simulink model "HQEV_MiL_20160830_integrate"  (Simulink 8.3)
settings: Solver=FixedStepDiscrete  StartTime=0.0  StopTime=inf  FixedStep=0.01  RelTol=1e-3
PostLoadFcn:
  | , if any(exist('dsrtsu_mdlpostloadfcn', 'file') == [2, 3, 6]), try dsrtsu_mdlpostloadfcn('Execute', bdroot); catch fprintf('Error in PostLoadFcn (dsrtsu_mdlpostloadfcn) for model "%s":\n %s\n', bdroot, lasterr); end, end,
values from neighbouring files (symbols this model uses):
  Bat_C_Ah = 36    [parameter_V1.mat]
  Bat_ocv_xIndex = [5 10 20 30 40 50 60 70 80 90 95]    [parameter_V1.mat]
  Bat_ocv_z = [329 332 340 345 347 351 358 372 377 386 391]    [parameter_V1.mat]
  Bat_R_ohm_z = [4.41 3.46 1.57 1.07 0.76 0.63 0.55 0.44 0.41 0.4 0.4 3.14 ... (66 elements, 11x6)]    [parameter_V1.mat]
  Bat_SOC_Init = 90    [parameter_V1.mat]
  Env_hum_pct_Ambient = 30    [parameter_V1.mat]
  Env_Slope_deg = 0    [parameter_V1.mat]
  Env_Temp_degC_Ambient = 25    [parameter_V1.mat]
  Env_v_kmph_HWind = 0    [parameter_V1.mat]
  Reducer_F_i = 7.23    [parameter_V1.mat]
  Reducer_R_i = 7.23    [parameter_V1.mat]
  Veh =     [parameter_V1.mat]
  Veh_A_m2_Fr = 2.246    [parameter_V1.mat]
  Veh_F_Brake =     [parameter_V1.mat]
  Veh_fac_AirDrag = 0.326    [parameter_V1.mat]
  Veh_fac_WhDragFrict_0 = 0.011    [parameter_V1.mat]
  Veh_g_mps2_C = 9.81    [parameter_V1.mat]
  Veh_GainBrake =     [parameter_V1.mat]
  Veh_h_m_COGHigh = 0.5    [parameter_V1.mat]
  Veh_J_kgm2_Wh = 1.3635    [parameter_V1.mat]
  Veh_L_m_AxlBas = 2.63    [parameter_V1.mat]
  Veh_M_kg = 1427    [parameter_V1.mat]
  Veh_mu_Brake = 0.4    [parameter_V1.mat]
  Veh_mu_Tyre =     [parameter_V1.mat]
  Veh_num_FrictPair = 8    [parameter_V1.mat]
  Veh_pct_Brk = 70    [parameter_V1.mat]
  Veh_r_dyn =     [parameter_V1.mat]
  Veh_r_m_BrkDisk = 0.136    [parameter_V1.mat]
  Veh_rho_kgpm3_Air = 1.2258    [parameter_V1.mat]
undefined symbols (not defined in the file or in its folder): DiscIntNeverNeededParam, p_bool_False_M, p_bool_True_M
libraries: BaseOperationLib_Browser x38, simulink x9, DTQC_lib x1, ERR_lib x1, MQM_lib x1, PTCL_lib x1, PUD_lib x1, TQD_lib x1, TQR_lib x1, VMM_lib x1, ACCA_lib x1, BBCA_lib x1
(part 10 of 15)

== system HQEV_MiL_20160830_integrate/MiL/Test_Integration/HCU/HCU/HCU/EVManager/evm_core ==
  Bus_hw_prep : Inport
  Bus_hw_algo : Inport  Port=2
  Bus Creator1 : BusCreator  Inputs=7
  DTQC : Subsystem
  ERR : Subsystem
  MQM : Subsystem
  PTCL : Subsystem
  PUD : Subsystem
  TQD : Subsystem
  TQR : Subsystem
  VMM : Subsystem
  Bus_evm_core : Outport
  wires:
  ERR/1(Bus_ERR) -> VMM/4(Bus_ERR)
  TQD/1(Bus_TQD) -> Bus Creator1/5, DTQC/1(Bus_TQD)
  TQR/1(Bus_TQR) -> Bus Creator1/4, TQD/1(Bus_TQR)
  PTCL/1(Bus_PTCL) -> Bus Creator1/3, TQR/1(Bus_PTCL)
  VMM/1(Bus_VMM) -> Bus Creator1/1, PUD/3(Bus_VMM)
  PUD/1(Bus_PUD) -> Bus Creator1/2, VMM/3(Bus_PUD)
  Bus_hw_algo/1 -> DTQC/3(Bus_hw_algo), MQM/3(Bus_hw_algo), TQD/3(Bus_hw_algo), TQR/3(Bus_hw_algo), PUD/2(Bus_hw_algo), ERR/2(Bus_hw_algo), VMM/2(Bus_hw_algo)
  Bus_hw_prep/1 -> DTQC/2(Bus_hw_prep), MQM/2(Bus_hw_prep), TQD/2(Bus_hw_prep), TQR/2(Bus_hw_prep), PTCL/1(Bus_hw_prep), PUD/1(Bus_hw_prep), ERR/1(Bus_hw_prep), VMM/1(Bus_hw_prep)
  Bus Creator1/1 -> Bus_evm_core/1  "Bus_evm_core"
  DTQC/1(Bus_DTQC) -> Bus Creator1/6, MQM/1(Bus_DTQC)
  MQM/1(Bus_MQM) -> Bus Creator1/7

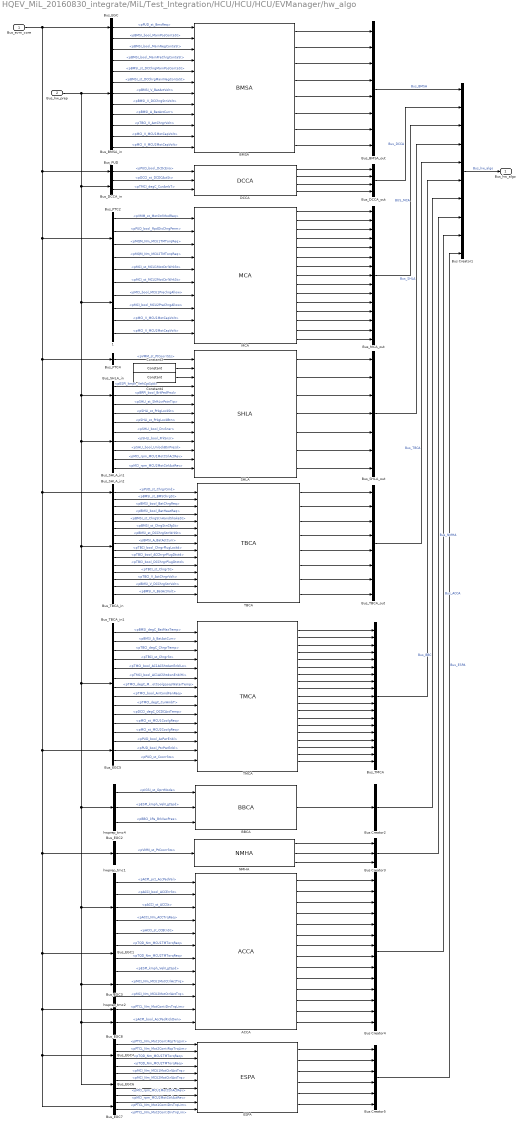
== system HQEV_MiL_20160830_integrate/MiL/Test_Integration/HCU/HCU/HCU/EVManager/hw_algo ==
  Bus_evm_core : Inport
  Bus_hw_prep : Inport  Port=2
  " 1" : BusSelector  OutputSignals=Bus_MCI.pMCI_st_MCU1MotCtrlWrkSt,Bus_MCI.pMCI_st_MCU2MotCtrlWrkSt,Bus_MCI.pMCI_bool_MCU1PrechrgAllow,Bus_MCI.pMCI_bool_MCU2PreChrgAllow,Bus_MCI.pMCI_V_MCU1MotCapVolt,Bus_MCI.pMCI_V_MCU2MotCapVolt
  ACCA : ACCA_lib/ACCA  SystemSampleTime=-1
  BBCA : BBCA_lib/BBCA  SystemSampleTime=-1
  BMSA : BMSA_lib/BMSA  SystemSampleTime=-1
  Bus Creator1 : BusCreator  Inputs=10
  Bus Creator2 : BusCreator  Inputs=1
  Bus Creator3 : BusCreator  Inputs=3
  Bus Creator4 : BusCreator  Inputs=14
  Bus Creator5 : BusCreator  Inputs=6
  Bus_BMSA_in : BusSelector  OutputSignals=Bus_BMSI.pBMSI_bool_MainPosContaSt,Bus_BMSI.pBMSI_bool_MainNegContaSt,Bus_BMSI.pBMSI_bool_MainPreChrgContaSt,Bus_BMSI.pBMSI_st_DCChrgMainPosContaSt,Bus_BMSI.pBMSI_st_DCChrgMainNegContaSt,Bus_BMSI.pBMSI_V_BatActVolt,Bus_BMSI.pBMSI_V_DCChrgStnVolt,Bus_BMSI.pBMSI_A_BatActCurr,Bus_TBCI.pTBCI_V_ActChrgrVolt,Bus_MCI.pMCI_V_MCU1MotCapVolt,Bus_MCI.pMCI_V_MCU2MotCapVolt
  Bus_BMSA_out : BusCreator  Inputs=8
  Bus_DCCA_in : BusSelector  OutputSignals=Bus_DCCI.pDCCI_st_DCDCActSt,Bus_TMCI.pTMCI_degC_CurAmbT
  Bus_DCCA_out : BusCreator
  Bus_EGC : BusSelector  OutputSignals=Bus_PUD.pPUD_st_BmsReq
  Bus_EGC1 : BusSelector  OutputSignals=Bus_TQD.pTQD_Nm_MCU1TMTorqReq,Bus_TQD.pTQD_Nm_MCU2TMTorqReq
  Bus_EGC2 : BusSelector  OutputSignals=Bus_VMM.pVMM_st_PtCoorrSts
  Bus_EGC3 : BusSelector  OutputSignals=Bus_PTCL.pPTCL_Nm_MotContiDrvTrqLim
  Bus_EGC4 : BusSelector  OutputSignals=Bus_PTCL.pPTCL_Nm_Mot1ContiRcpTrqLim,Bus_PTCL.pPTCL_Nm_Mot2ContiRcpTrqLim,Bus_TQD.pTQD_Nm_MCU1TMTorqReq,Bus_TQD.pTQD_Nm_MCU2TMTorqReq
  Bus_EGC5 : BusSelector  OutputSignals=Bus_PUD.pPUD_bool_AcPwrEnbl,Bus_PUD.pPUD_bool_PtcPwrEnbl,Bus_PUD.pPUD_st_CoorrSts
  Bus_EGC6 : BusSelector  OutputSignals=Bus_MCI.pMCI_Nm_MCU1MotCtrlActTrq,Bus_MCI.pMCI_Nm_MCU2MotCtrlActTrq,Bus_MCI.pMCI_rpm_MCU1MotCtrlActRev,Bus_MCI.pMCI_rpm_MCU2MotCtrlActRev
  Bus_EGC7 : BusSelector  OutputSignals=Bus_PTCL.pPTCL_Nm_Mot1ContiDrvTrqLim,Bus_PTCL.pPTCL_Nm_Mot2ContiDrvTrqLim
  Bus_EGC8 : BusSelector  OutputSignals=Bus_ACPI.pACPI_bool_AccPedKickDwn
  Bus_MCA_out : BusCreator  Inputs=15
  Bus_PTC2 : BusSelector  OutputSignals=Bus_VMM.pVMM_st_MotCtrlModReq,Bus_PUD.pPUD_bool_RpdDisChrgPerm,Bus_MQM.pMQM_Nm_MCU1TMTorqReq,Bus_MQM.pMQM_Nm_MCU2TMTorqReq
  Bus_PTC4 : BusSelector  OutputSignals=Bus_VMM.pVMM_st_PtCoorrSts
  Bus_PUD : BusSelector  OutputSignals=Bus_PUD.pPUD_bool_DcDcEna
  Bus_SHLA_in : BusSelector  OutputSignals=Bus_ESPI.pESPI_kmph_VehLgtSpd,Bus_BRPI.pBRPI_bool_BrkPedPrsd,Bus_SHLI.pSHLI_st_ShftLvrPstnTip
  Bus_SHLA_in1 : BusSelector  OutputSignals=Bus_SHLI.pSHLI_st_PrkgLockSt,Bus_SHLI.pSHLI_st_PrkgLockBtn,Bus_SHLI.pSHLI_bool_DrvSnsr,Bus_SHLI.pSHLI_bool_PrkSnsr,Bus_SHLI.pSHLI_bool_UnlockBtnPresd,Bus_MCI.pMCI_rpm_MCU1MotCtrlActRev,Bus_MCI.pMCI_rpm_MCU2MotCtrlActRev
  Bus_SHLA_in2 : BusSelector  OutputSignals=Bus_PUD.pPUD_st_ChrgrCmd
  Bus_SHLA_out : BusCreator  Inputs=7
  Bus_TBCA_in : BusSelector  OutputSignals=Bus_BMSI.pBMSI_st_BMSChrgSt,Bus_BMSI.pBMSI_bool_BatChrgReq,Bus_BMSI.pBMSI_bool_BatHeatReq,Bus_BMSI.pBMSI_st_ChrgStnHandShakeSt,Bus_BMSI.pBMSI_st_ChrgStnCfgSt,Bus_BMSI.pBMSI_st_DCChrgStnWrkSt,Bus_BMSI.pBMSI_A_BatActCurr,Bus_TBCI.pTBCI_bool_ChrgrPlugLockd,Bus_TBCI.pTBCI_bool_ACChrgrPlugDtctd,Bus_TBCI.pTBCI_bool_DCChrgrPlugDtctd,Bus_TBCI.pTBCI_st_ChrgrSt,Bus_TBCI.pTBCI_V_ActChrgrVolt,Bus_BMSI.pBMSI_V_DCChrgStnVolt,Bus_BMSI.pBMSI_V_BatActVolt
  Bus_TBCA_in1 : BusSelector  OutputSignals=Bus_BMSI.pBMSI_degC_BatMaxTemp,Bus_BMSI.pBMSI_A_BatActCurr,Bus_TBCI.pTBCI_degC_ChrgrTemp,Bus_TBCI.pTBCI_st_ChrgrSt,Bus_TMCI.pTMCI_bool_AC1ACShtdwnEnblLo,Bus_TMCI.pTMCI_bool_AC1ACShtdwnEnblHi,Bus_TMCI.pTMCI_degC_MotCoolgLoopWaterTemp,Bus_TMCI.pTMCI_bool_AirCondFanReq,Bus_TMCI.pTMCI_degC_CurAmbT,Bus_DCCI.pDCCI_degC_DCDCActTemp,Bus_MCI.pMCI_st_MCU1CoolgReq,Bus_MCI.pMCI_st_MCU2CoolgReq
  Bus_TBCA_out : BusCreator  Inputs=8
  Bus_TMCA : BusCreator  Inputs=19
  Constant3 : BaseOperationLib_Browser/Sources&Sinks/Constant  Value=p_bool_True_M  OutMin=[]  OutMax=[]  OutDataTypeMode=boolean  OutDataType=fixdt(1, 16)  ConRadixGroup=Use specified scaling  OutScaling=2^0  OutDataTypeStr=boolean
  Constant4 : BaseOperationLib_Browser/Sources&Sinks/Constant  Value=p_bool_False_M  OutMin=[]  OutMax=[]  OutDataTypeMode=boolean  OutDataType=fixdt(1, 16)  ConRadixGroup=Use specified scaling  OutScaling=2^0  OutDataTypeStr=boolean
  DCCA : DCCA_lib/DCCA  SystemSampleTime=-1
  ESPA : ESPA_lib/ESPA  SystemSampleTime=-1
  MCA : MCA_lib/MCA  SystemSampleTime=-1
  NMHA : NMHA_lib/NMHA  SystemSampleTime=-1
  SHLA : SHLA_lib/SHLA  SystemSampleTime=-1
  TBCA : TBCA_lib/TBCA  SystemSampleTime=-1
  TMCA : TMCA_lib/TMCA  SystemSampleTime=-1
  hwprep_tmc1 : BusSelector  OutputSignals=Bus_ACPI.pACPI_pct_AccPedVal,Bus_ACCI.pACCI_bool_ACCErrSt,Bus_ACCI.pACCI_st_ACCSt,Bus_ACCI.pACCI_Nm_ACCTrqReq,Bus_ACCI.pACCI_st_CCBtnSt
  hwprep_tmc2 : BusSelector  OutputSignals=Bus_ESPI.pESPI_kmph_VehLgtSpd,Bus_MCI.pMCI_Nm_MCU1MotCtrlActTrq,Bus_MCI.pMCI_Nm_MCU2MotCtrlActTrq
  hwprep_tmc4 : BusSelector  OutputSignals=Bus_IGSI.pIGSI_st_OprtMode,Bus_ESPI.pESPI_kmph_VehLgtSpd,Bus_BBCI.pBBCI_kPa_BrkVacPres
  Bus_hw_algo : Outport
  wires:
  Bus_BMSA_in/8 -> BMSA/9  "<pBMSI_A_BatActCurr>"
  MCA/15 -> Bus_MCA_out/15
  MCA/14 -> Bus_MCA_out/14
  MCA/13 -> Bus_MCA_out/13
  MCA/12 -> Bus_MCA_out/12
  MCA/11 -> Bus_MCA_out/11
  MCA/10 -> Bus_MCA_out/10
  MCA/9 -> Bus_MCA_out/9
  MCA/8 -> Bus_MCA_out/8
  MCA/7 -> Bus_MCA_out/7
  MCA/6 -> Bus_MCA_out/6
  MCA/5 -> Bus_MCA_out/5
  MCA/4 -> Bus_MCA_out/4
  MCA/3 -> Bus_MCA_out/3
  MCA/2 -> Bus_MCA_out/2
  MCA/1 -> Bus_MCA_out/1
  DCCA/1 -> Bus_DCCA_out/1
  Bus_DCCA_in/1 -> DCCA/2  "<pDCCI_st_DCDCActSt>"
  Bus_PUD/1 -> DCCA/1  "<pPUD_bool_DcDcEna>"
  DCCA/2 -> Bus_DCCA_out/2
  DCCA/3 -> Bus_DCCA_out/3
  DCCA/4 -> Bus_DCCA_out/4
  Bus_DCCA_in/2 -> DCCA/3  "<pTMCI_degC_CurAmbT>"
  Bus_DCCA_out/1 -> Bus Creator1/2  "Bus_DCCA"
  Constant4/1 -> SHLA/3
  Constant3/1 -> SHLA/2
  Bus_SHLA_in1/7 -> SHLA/13  "<pMCI_rpm_MCU2MotCtrlActRev>"
  Bus_SHLA_in1/6 -> SHLA/12  "<pMCI_rpm_MCU1MotCtrlActRev>"
  Bus_PTC2/2 -> MCA/2  "<pPUD_bool_RpdDisChrgPerm>"
  SHLA/7 -> Bus_SHLA_out/7
  SHLA/6 -> Bus_SHLA_out/6
  SHLA/5 -> Bus_SHLA_out/5
  SHLA/4 -> Bus_SHLA_out/4
  SHLA/3 -> Bus_SHLA_out/3
  SHLA/2 -> Bus_SHLA_out/2
  SHLA/1 -> Bus_SHLA_out/1
  Bus_SHLA_in1/5 -> SHLA/11  "<pSHLI_bool_UnlockBtnPresd>"
  Bus_SHLA_in/3 -> SHLA/6  "<pSHLI_st_ShftLvrPstnTip>"
  Bus_SHLA_in/2 -> SHLA/5  "<pBRPI_bool_BrkPedPrsd>"
  Bus_SHLA_in/1 -> SHLA/4  "<pESPI_kmph_VehLgtSpd>"
  Bus_TBCA_in/13 -> TBCA/14  "<pBMSI_V_DCChrgStnVolt>"
  Bus_TBCA_in/12 -> TBCA/13  "<pTBCI_V_ActChrgrVolt>"
  Bus Creator3/1 -> Bus Creator1/8  "Bus_NMHA"
  NMHA/3 -> Bus Creator3/3
  NMHA/2 -> Bus Creator3/2
  NMHA/1 -> Bus Creator3/1
  Bus_EGC2/1 -> NMHA/1  "<pVMM_st_PtCoorrSts>"
  Bus_PTC2/4 -> MCA/4  "<pMQM_Nm_MCU2TMTorqReq>"
  Bus_PTC2/3 -> MCA/3  "<pMQM_Nm_MCU1TMTorqReq>"
  Bus_PTC2/1 -> MCA/1  "<pVMM_st_MotCtrlModReq>"
  Bus_TBCA_in/7 -> TBCA/8  "<pBMSI_A_BatActCurr>"
  BMSA/8 -> Bus_BMSA_out/8
  BMSA/7 -> Bus_BMSA_out/7
  BMSA/6 -> Bus_BMSA_out/6
  BMSA/5 -> Bus_BMSA_out/5
  BMSA/4 -> Bus_BMSA_out/4
  BMSA/3 -> Bus_BMSA_out/3
  BMSA/2 -> Bus_BMSA_out/2
  BMSA/1 -> Bus_BMSA_out/1
  Bus_BMSA_in/11 -> BMSA/12  "<pMCI_V_MCU2MotCapVolt>"
  Bus_BMSA_in/10 -> BMSA/11  "<pMCI_V_MCU1MotCapVolt>"
  Bus_BMSA_in/9 -> BMSA/10  "<pTBCI_V_ActChrgrVolt>"
  Bus_BMSA_in/7 -> BMSA/8  "<pBMSI_V_DCChrgStnVolt>"
  hwprep_tmc4/3 -> BBCA/3  "<pBBCI_kPa_BrkVacPres>"
  Bus Creator2/1 -> Bus Creator1/7  "Bus_BBC"
  hwprep_tmc4/1 -> BBCA/1  "<pIGSI_st_OprtMode>"
  hwprep_tmc4/2 -> BBCA/2  "<pESPI_kmph_VehLgtSpd>"
  BBCA/1 -> Bus Creator2/1
  Bus_MCA_out/1 -> Bus Creator1/3  "BUS_MCA"
  " 1"/6 -> MCA/10  "<pMCI_V_MCU2MotCapVolt>"
  " 1"/5 -> MCA/9  "<pMCI_V_MCU1MotCapVolt>"
  " 1"/1 -> MCA/5  "<pMCI_st_MCU1MotCtrlWrkSt>"
  " 1"/4 -> MCA/8  "<pMCI_bool_MCU2PreChrgAllow>"
  " 1"/3 -> MCA/7  "<pMCI_bool_MCU1PrechrgAllow>"
  " 1"/2 -> MCA/6  "<pMCI_st_MCU2MotCtrlWrkSt>"
  Bus_TBCA_in/11 -> TBCA/12  "<pTBCI_st_ChrgrSt>"
  TBCA/8 -> Bus_TBCA_out/8
  Bus_EGC/1 -> BMSA/1  "<pPUD_st_BmsReq>"
  Bus_BMSA_in/6 -> BMSA/7  "<pBMSI_V_BatActVolt>"
  Bus_BMSA_in/5 -> BMSA/6  "<pBMSI_st_DCChrgMainNegContaSt>"
  Bus_BMSA_in/4 -> BMSA/5  "<pBMSI_st_DCChrgMainPosContaSt>"
  Bus_BMSA_in/3 -> BMSA/4  "<pBMSI_bool_MainPreChrgContaSt>"
  Bus_BMSA_in/2 -> BMSA/3  "<pBMSI_bool_MainNegContaSt>"
  Bus_BMSA_in/1 -> BMSA/2  "<pBMSI_bool_MainPosContaSt>"
  Bus_TBCA_in/10 -> TBCA/11  "<pTBCI_bool_DCChrgrPlugDtctd>"
  Bus_TBCA_in/9 -> TBCA/10  "<pTBCI_bool_ACChrgrPlugDtctd>"
  Bus_TBCA_in/8 -> TBCA/9  "<pTBCI_bool_ChrgrPlugLockd>"
  Bus_TBCA_in/6 -> TBCA/7  "<pBMSI_st_DCChrgStnWrkSt>"
  Bus_TBCA_in/5 -> TBCA/6  "<pBMSI_st_ChrgStnCfgSt>"
  Bus_TBCA_in/4 -> TBCA/5  "<pBMSI_st_ChrgStnHandShakeSt>"
  Bus_TBCA_in/3 -> TBCA/4  "<pBMSI_bool_BatHeatReq>"
  Bus_TBCA_in/2 -> TBCA/3  "<pBMSI_bool_BatChrgReq>"
  Bus_TBCA_in/1 -> TBCA/2  "<pBMSI_st_BMSChrgSt>"
  Bus_SHLA_in2/1 -> TBCA/1  "<pPUD_st_ChrgrCmd>"
  TBCA/7 -> Bus_TBCA_out/7
  TBCA/6 -> Bus_TBCA_out/6
  TBCA/5 -> Bus_TBCA_out/5
  TBCA/4 -> Bus_TBCA_out/4
  TBCA/3 -> Bus_TBCA_out/3
  TBCA/2 -> Bus_TBCA_out/2
  TBCA/1 -> Bus_TBCA_out/1
  Bus Creator1/1 -> Bus_hw_algo/1  "Bus_hw_algo"
  Bus_hw_prep/1 -> Bus_SHLA_in/1, Bus_SHLA_in1/1, Bus_TBCA_in1/1, hwprep_tmc4/1, hwprep_tmc1/1, hwprep_tmc2/1, Bus_EGC6/1, Bus_EGC8/1, Bus_TBCA_in/1, " 1"/1, Bus_DCCA_in/1, Bus_BMSA_in/1
  Bus_evm_core/1 -> Bus_PTC4/1, Bus_EGC5/1, Bus_EGC2/1, Bus_EGC1/1, Bus_EGC3/1, Bus_EGC4/1, Bus_EGC7/1, Bus_SHLA_in2/1, Bus_PTC2/1, Bus_PUD/1, Bus_EGC/1
  Bus_BMSA_out/1 -> Bus Creator1/1  "Bus_BMSA"
  Bus_SHLA_out/1 -> Bus Creator1/4  "Bus_SHLA"
  Bus_TBCA_out/1 -> Bus Creator1/5  "Bus_TBCA"
  Bus_SHLA_in1/1 -> SHLA/7  "<pSHLI_st_PrkgLockSt>"
  Bus_SHLA_in1/2 -> SHLA/8  "<pSHLI_st_PrkgLockBtn>"
  Bus_SHLA_in1/3 -> SHLA/9  "<pSHLI_bool_DrvSnsr>"
  Bus_SHLA_in1/4 -> SHLA/10  "<pSHLI_bool_PrkSnsr>"
  Bus_PTC4/1 -> SHLA/1  "<pVMM_st_PtCoorrSts>"
  Bus_TBCA_in/14 -> TBCA/15  "<pBMSI_V_BatActVolt>"
  TMCA/19 -> Bus_TMCA/19
  TMCA/18 -> Bus_TMCA/18
  TMCA/17 -> Bus_TMCA/17
  TMCA/16 -> Bus_TMCA/16
  TMCA/15 -> Bus_TMCA/15
  TMCA/14 -> Bus_TMCA/14
  TMCA/13 -> Bus_TMCA/13
  TMCA/12 -> Bus_TMCA/12
  TMCA/11 -> Bus_TMCA/11
  TMCA/10 -> Bus_TMCA/10
  TMCA/9 -> Bus_TMCA/9
  TMCA/8 -> Bus_TMCA/8
  TMCA/7 -> Bus_TMCA/7
  TMCA/6 -> Bus_TMCA/6
  TMCA/5 -> Bus_TMCA/5
  TMCA/4 -> Bus_TMCA/4
  TMCA/3 -> Bus_TMCA/3
  TMCA/2 -> Bus_TMCA/2
  TMCA/1 -> Bus_TMCA/1
  Bus_EGC5/3 -> TMCA/15  "<pPUD_st_CoorrSts>"
  Bus_EGC5/2 -> TMCA/14  "<pPUD_bool_PtcPwrEnbl>"
  Bus_EGC5/1 -> TMCA/13  "<pPUD_bool_AcPwrEnbl>"
  Bus_TBCA_in1/12 -> TMCA/12  "<pMCI_st_MCU2CoolgReq>"
  Bus_TBCA_in1/11 -> TMCA/11  "<pMCI_st_MCU1CoolgReq>"
  Bus_TBCA_in1/10 -> TMCA/10  "<pDCCI_degC_DCDCActTemp>"
  Bus_TBCA_in1/9 -> TMCA/9  "<pTMCI_degC_CurAmbT>"
  Bus_TBCA_in1/8 -> TMCA/8  "<pTMCI_bool_AirCondFanReq>"
  Bus_TBCA_in1/7 -> TMCA/7  "<pTMCI_degC_MotCoolgLoopWaterTemp>"
  Bus_TBCA_in1/6 -> TMCA/6  "<pTMCI_bool_AC1ACShtdwnEnblHi>"
  Bus_TBCA_in1/5 -> TMCA/5  "<pTMCI_bool_AC1ACShtdwnEnblLo>"
  Bus_TBCA_in1/4 -> TMCA/4  "<pTBCI_st_ChrgrSt>"
  Bus_TBCA_in1/3 -> TMCA/3  "<pTBCI_degC_ChrgrTemp>"
  Bus_TBCA_in1/2 -> TMCA/2  "<pBMSI_A_BatActCurr>"
  Bus_TBCA_in1/1 -> TMCA/1  "<pBMSI_degC_BatMaxTemp>"
  Bus_TMCA/1 -> Bus Creator1/6
  ACCA/1 -> Bus Creator4/1
  ACCA/2 -> Bus Creator4/2
  ACCA/3 -> Bus Creator4/3
  ACCA/4 -> Bus Creator4/4
  ACCA/5 -> Bus Creator4/5
  ACCA/6 -> Bus Creator4/6
  ACCA/7 -> Bus Creator4/7
  ACCA/8 -> Bus Creator4/8
  ACCA/9 -> Bus Creator4/9
  ACCA/10 -> Bus Creator4/10
  ACCA/11 -> Bus Creator4/11
  ACCA/12 -> Bus Creator4/12
  hwprep_tmc1/1 -> ACCA/1  "<pACPI_pct_AccPedVal>"
  hwprep_tmc1/2 -> ACCA/2  "<pACCI_bool_ACCErrSt>"
  hwprep_tmc1/3 -> ACCA/3  "<pACCI_st_ACCSt>"
  hwprep_tmc1/4 -> ACCA/4  "<pACCI_Nm_ACCTrqReq>"
  hwprep_tmc1/5 -> ACCA/5  "<pACCI_st_CCBtnSt>"
  hwprep_tmc2/1 -> ACCA/8  "<pESPI_kmph_VehLgtSpd>"
  hwprep_tmc2/2 -> ACCA/9  "<pMCI_Nm_MCU1MotCtrlActTrq>"
  hwprep_tmc2/3 -> ACCA/10  "<pMCI_Nm_MCU2MotCtrlActTrq>"
  Bus_EGC3/1 -> ACCA/11  "<pPTCL_Nm_MotContiDrvTrqLim>"
  Bus Creator4/1 -> Bus Creator1/9  "Bus_ACCA"
  ESPA/1 -> Bus Creator5/1
  ESPA/2 -> Bus Creator5/2
  ESPA/3 -> Bus Creator5/3
  ESPA/4 -> Bus Creator5/4
  Bus Creator5/1 -> Bus Creator1/10  "Bus_ESPA"
  Bus_EGC6/1 -> ESPA/5  "<pMCI_Nm_MCU1MotCtrlActTrq>"
  Bus_EGC6/2 -> ESPA/6  "<pMCI_Nm_MCU2MotCtrlActTrq>"
  Bus_EGC6/3 -> ESPA/7  "<pMCI_rpm_MCU1MotCtrlActRev>"
  Bus_EGC6/4 -> ESPA/8  "<pMCI_rpm_MCU2MotCtrlActRev>"
  ACCA/13 -> Bus Creator4/13
  ESPA/5 -> Bus Creator5/5
  ESPA/6 -> Bus Creator5/6
  Bus_EGC7/1 -> ESPA/9  "<pPTCL_Nm_Mot1ContiDrvTrqLim>"
  Bus_EGC7/2 -> ESPA/10  "<pPTCL_Nm_Mot2ContiDrvTrqLim>"
  Bus_EGC4/1 -> ESPA/1  "<pPTCL_Nm_Mot1ContiRcpTrqLim>"
  Bus_EGC4/2 -> ESPA/2  "<pPTCL_Nm_Mot2ContiRcpTrqLim>"
  Bus_EGC4/3 -> ESPA/3  "<pTQD_Nm_MCU1TMTorqReq>"
  Bus_EGC4/4 -> ESPA/4  "<pTQD_Nm_MCU2TMTorqReq>"
  Bus_EGC8/1 -> ACCA/12  "<pACPI_bool_AccPedKickDwn>"
  ACCA/14 -> Bus Creator4/14
  Bus_EGC1/1 -> ACCA/6  "<pTQD_Nm_MCU1TMTorqReq>"
  Bus_EGC1/2 -> ACCA/7  "<pTQD_Nm_MCU2TMTorqReq>"

== system HQEV_MiL_20160830_integrate/MiL/Test_Integration/HCU/HCU/HCU/EVManager/hw_post ==
  Bus_evm_core : Inport
  Bus_hw_algo : Inport  Port=2
  Bus_hw_prep : Inport  Port=3
  Bus Selector1 : BusSelector  OutputSignals=Bus_BMSA.pBMSA_bool_MaiPosContaCmd,Bus_BMSA.pBMSA_bool_MaiNegContaCmd,Bus_BMSA.pBMSA_bool_MaiPrecContaCmd,Bus_BMSA.pBMSA_bool_DCChrgNegContaCmd,Bus_BMSA.pBMSA_bool_DCChrgPosContaCmd,Bus_TBCA.pTBCA_bool_BatChrgPerm,Bus_TBCA.pTBCA_bool_BatHeatPerm,Bus_DCCA.pDCCA_bool_DcDcCmd,Bus_DCCA.pDCCA_V_DcDcOutUSp
  Bus Selector11 : BusSelector  OutputSignals=Bus_BMSI.pBMSI_st_BatIslaMeasSt,Bus_DCCI.pDCCI_st_DCDCActSt,Bus_BMSI.pBMSI_degC_BatAvgTemp,Bus_BMSI.pBMSI_st_BMSErr,Bus_BMSI.pBMSI_min_RemainChrgTime,Bus_BMSI.pBMSI_kw_InstnsPwrCnsmp,Bus_BMSI.pBMSI_V_BatActVolt
  Bus Selector12 : BusSelector  OutputSignals=Bus_VMM.pVMM_st_PtCoorrSts
  Bus Selector15 : BusSelector  OutputSignals=Bus_ESPI.pESPI_kmph_VehLgtSpd,Bus_TBCI.pTBCI_bool_ACChrgrPlugDtctd,Bus_TBCI.pTBCI_bool_DCChrgrPlugDtctd,Bus_ARBI.pARBI_st_StCrash
  Bus Selector19 : BusSelector  OutputSignals=signal6.pTMCA_bool_RemainACOnTip,Bus_NMHA.pNMHA_bool_CanSlpCmd,BUS_MCA.pMCA_Nm_MCU1TMTorqReq,BUS_MCA.pMCA_Nm_MCU2TMTorqReq
  Bus Selector2 : BusSelector  OutputSignals=Bus_ACPI.pACPI_pct_AccPedVal,Bus_BRPI.pBRPI_bool_BrkPedPrsd
  Bus Selector3 : BusSelector  OutputSignals=Bus_ACCA.pACCA_bool_KickDwnReq,Bus_ACCA.pACCA_bool_AccelPedOvrid,Bus_ACCA.pACCA_pct_CalcAccelPedPstn,Bus_ACCA.pACCA_bool_RespACC,Bus_ACCA.pACCA_bool_CCMainSwt,Bus_ACCA.pACCA_bool_CCCancelSwt,Bus_ACCA.pACCA_bool_CCSetOrCoastSwt,Bus_ACCA.pACCA_bool_HeadwaySwt,Bus_ACCA.pACCA_bool_CCSwtErr,Bus_ACCA.pACCA_bool_CCRsmOrAccelSwt,Bus_ACCA.pACCA_Nm_ActDrvReqTrq,Bus_ACCA.pACCA_Nm_MotMaxDrvTrq,Bus_ACCA.pACCA_Nm_IndicateDrvPrimTrq,Bus_ACCA.pACCA_Nm_IndicateDrvSecTrq
  Bus Selector30 : BusSelector  OutputSignals=Bus_VMM.pVMM_st_PtCoorrSts
  Bus Selector32 : BusSelector  OutputSignals=Bus_BMSI.pBMSI_A_BatActCurr,Bus_TBCI.pTBCI_bool_ACChrgrPlugDtctd,Bus_TBCI.pTBCI_bool_DCChrgrPlugDtctd,Bus_BMSI.pBMSI_st_BMSChrgSt,Bus_BMSI.pBMSI_pct_BatSOC,Bus_SHLI.pSHLI_st_ECOSwtSt,Bus_IGSI.pIGSI_st_OprtMode,Bus_MCI.pMCI_Nm_MCU1MotCtrlActTrq,Bus_MCI.pMCI_rpm_MCU1MotCtrlActRev,Bus_MCI.pMCI_rpm_MCU2MotCtrlActRev,Bus_DCCI.pDCCI_V_DCDCOutVolt
  Bus Selector33 : BusSelector  OutputSignals=BUS_MCA.pMCA_Nm_MCU1TMTorqReq,BUS_MCA.pMCA_bool_MCU1MotRpdDchaReq,BUS_MCA.pMCA_st_MCU1MotCtlrStModReq,BUS_MCA.pMCA_bool_MCU1AntijerkOffReq,BUS_MCA.pMCA_bool_MCU1StopReqToMCU,BUS_MCA.pMCA_Nm_MCU2TMTorqReq,BUS_MCA.pMCA_bool_MCU2MotRpdDchaReq,BUS_MCA.pMCA_st_MCU2MotCtlrStModReq,BUS_MCA.pMCA_bool_MCU2AntijerkOffReq,BUS_MCA.pMCA_bool_MCU2StopReqToMCU,Bus_NMHA.pNMHA_bool_CanSlpCmd
  Bus Selector34 : BusSelector  OutputSignals=Bus_BBC.pBBCA_bool_BrkVacPmpCmd,signal6.pTMCA_pct_PtcCtrlCmd,signal6.pTMCA_bool_HiSpdFanCmd,signal6.pTMCA_bool_LoSpdFanCmd,signal6.pTMCA_pct_Mot1WtrPmpCmd,signal6.pTMCA_pct_BatWtrPmpCmd,signal6.pTMCA_pct_Mot2WtrPmpCmd,BUS_MCA.pMCA_bool_MotVirtIgOn,Bus_NMHA.pNMHA_bool_MaiRlyCtlCmd,Bus_NMHA.pNMHA_bool_VCUSleep,signal6.pTMCA_bool_ChargerValve1CtrlB,signal6.pTMCA_bool_ChargerValve1CtrlC,signal6.pTMCA_bool_RMotorValve2CtrlB,signal6.pTMCA_bool_RMotorValve2CtrlC
  Bus Selector4 : BusSelector  OutputSignals=Bus_ESPA.pESPA_Nm_MCU1ActBrkTrq,Bus_ESPA.pESPA_Nm_MCU1MaxDrvTrq,Bus_ESPA.pESPA_Nm_MCU1MaxGenrTrq,Bus_ESPA.pESPA_Nm_MCU2ActBrkTrq,Bus_ESPA.pESPA_Nm_MCU2MaxDrvTrq,Bus_ESPA.pESPA_Nm_MCU2MaxGenrTrq
  Bus Selector5 : BusSelector  OutputSignals=signal6.pTMCA_bool_VechPermit,signal6.pTMCA_bool_IGOffReq,signal6.pTMCA_bool_AirCdnCmd,signal6.pTMCA_bool_BatCoolgReq,Bus_SHLA.pSHLA_st_ShftLvrPosnIC,Bus_SHLA.pSHLA_st_PrkgLock
  Bus Selector6 : BusSelector  OutputSignals=Bus_ESPI.pESPI_ratio_AltitudeFac
  CAN_EV : CAN_EV_lib/CAN_EV  SystemSampleTime=-1
  CAN_PT : CAN_PT_lib/CAN_PT  SystemSampleTime=-1
  HWO : HWO_lib/HWO  SystemSampleTime=-1
  bus_CAN_EV : BusCreator  Inputs=24
  bus_CAN_PT : BusCreator  Inputs=63
  bus_HWO : BusCreator  Inputs=14
  bus_in5 : BusCreator  Inputs=3
  Bus_RTE_out : Outport
  wires:
  Bus Selector34/10 -> HWO/10  "<pNMHA_bool_VCUSleep>"
  CAN_EV/24 -> bus_CAN_EV/24
  Bus Selector33/11 -> CAN_EV/11  "<pNMHA_bool_CanSlpCmd>"
  CAN_EV/23 -> bus_CAN_EV/23
  CAN_EV/22 -> bus_CAN_EV/22
  CAN_EV/21 -> bus_CAN_EV/21
  CAN_EV/20 -> bus_CAN_EV/20
  CAN_EV/19 -> bus_CAN_EV/19
  CAN_EV/18 -> bus_CAN_EV/18
  Bus Selector15/4 -> CAN_EV/25  "<pARBI_st_StCrash>"
  Bus Selector34/1 -> HWO/1  "<pBBCA_bool_BrkVacPmpCmd>"
  bus_HWO/1 -> bus_in5/3  "HWO_BUS"
  HWO/14 -> bus_HWO/14
  HWO/13 -> bus_HWO/13
  HWO/12 -> bus_HWO/12
  HWO/11 -> bus_HWO/11
  HWO/10 -> bus_HWO/10
  HWO/9 -> bus_HWO/9
  HWO/8 -> bus_HWO/8
  HWO/7 -> bus_HWO/7
  HWO/6 -> bus_HWO/6
  HWO/5 -> bus_HWO/5
  HWO/4 -> bus_HWO/4
  HWO/3 -> bus_HWO/3
  HWO/2 -> bus_HWO/2
  HWO/1 -> bus_HWO/1
  Bus Selector34/14 -> HWO/14  "<pTMCA_bool_RMotorValve2CtrlC>"
  Bus Selector34/13 -> HWO/13  "<pTMCA_bool_RMotorValve2CtrlB>"
  Bus Selector34/12 -> HWO/12  "<pTMCA_bool_ChargerValve1CtrlC>"
  Bus Selector34/11 -> HWO/11  "<pTMCA_bool_ChargerValve1CtrlB>"
  Bus Selector34/2 -> HWO/2  "<pTMCA_pct_PtcCtrlCmd>"
  Bus Selector34/3 -> HWO/3  "<pTMCA_bool_HiSpdFanCmd>"
  Bus Selector34/4 -> HWO/4  "<pTMCA_bool_LoSpdFanCmd>"
  Bus Selector34/5 -> HWO/5  "<pTMCA_pct_Mot1WtrPmpCmd>"
  Bus Selector34/6 -> HWO/6  "<pTMCA_pct_BatWtrPmpCmd>"
  Bus Selector34/8 -> HWO/8  "<pMCA_bool_MotVirtIgOn>"
  Bus Selector34/7 -> HWO/7  "<pTMCA_pct_Mot2WtrPmpCmd>"
  Bus Selector34/9 -> HWO/9  "<pNMHA_bool_MaiRlyCtlCmd>"
  Bus Selector15/3 -> CAN_EV/24  "<pTBCI_bool_DCChrgrPlugDtctd>"
  Bus Selector15/2 -> CAN_EV/23  "<pTBCI_bool_ACChrgrPlugDtctd>"
  Bus_hw_prep/1 -> Bus Selector15/1, Bus Selector32/1, Bus Selector11/1, Bus Selector6/1, Bus Selector2/1
  Bus Selector15/1 -> CAN_EV/22  "<pESPI_kmph_VehLgtSpd>"
  Bus Selector12/1 -> CAN_EV/21  "<pVMM_st_PtCoorrSts>"
  Bus_evm_core/1 -> Bus Selector30/1, Bus Selector12/1
  Bus_hw_algo/1 -> Bus Selector19/1, Bus Selector3/1, Bus Selector34/1, Bus Selector4/1, Bus Selector5/1, Bus Selector1/1, Bus Selector33/1
  bus_in5/1 -> Bus_RTE_out/1  "Bus_RTE_out"
  bus_CAN_PT/1 -> bus_in5/2  "CAN_PT_BUS"
  bus_CAN_EV/1 -> bus_in5/1  "CAN_EV_BUS"
  CAN_EV/1 -> bus_CAN_EV/1
  CAN_EV/2 -> bus_CAN_EV/2
  CAN_EV/3 -> bus_CAN_EV/3
  CAN_EV/4 -> bus_CAN_EV/4
  CAN_EV/5 -> bus_CAN_EV/5
  CAN_EV/6 -> bus_CAN_EV/6
  CAN_EV/7 -> bus_CAN_EV/7
  CAN_EV/8 -> bus_CAN_EV/8
  CAN_EV/9 -> bus_CAN_EV/9
  CAN_EV/10 -> bus_CAN_EV/10
  CAN_EV/11 -> bus_CAN_EV/11
  CAN_EV/12 -> bus_CAN_EV/12
  CAN_EV/13 -> bus_CAN_EV/13
  CAN_EV/14 -> bus_CAN_EV/14
  CAN_EV/15 -> bus_CAN_EV/15
  CAN_EV/16 -> bus_CAN_EV/16
  CAN_EV/17 -> bus_CAN_EV/17
  Bus Selector33/1 -> CAN_EV/1  "<pMCA_Nm_MCU1TMTorqReq>"
  Bus Selector33/2 -> CAN_EV/2  "<pMCA_bool_MCU1MotRpdDchaReq>"
  Bus Selector33/3 -> CAN_EV/3  "<pMCA_st_MCU1MotCtlrStModReq>"
  Bus Selector33/4 -> CAN_EV/4  "<pMCA_bool_MCU1AntijerkOffReq>"
  Bus Selector33/5 -> CAN_EV/5  "<pMCA_bool_MCU1StopReqToMCU>"
  Bus Selector33/6 -> CAN_EV/6  "<pMCA_Nm_MCU2TMTorqReq>"
  Bus Selector33/7 -> CAN_EV/7  "<pMCA_bool_MCU2MotRpdDchaReq>"
  Bus Selector33/8 -> CAN_EV/8  "<pMCA_st_MCU2MotCtlrStModReq>"
  Bus Selector33/9 -> CAN_EV/9  "<pMCA_bool_MCU2AntijerkOffReq>"
  Bus Selector33/10 -> CAN_EV/10  "<pMCA_bool_MCU2StopReqToMCU>"
  Bus Selector1/1 -> CAN_EV/12  "<pBMSA_bool_MaiPosContaCmd>"
  Bus Selector1/2 -> CAN_EV/13  "<pBMSA_bool_MaiNegContaCmd>"
  Bus Selector1/3 -> CAN_EV/14  "<pBMSA_bool_MaiPrecContaCmd>"
  Bus Selector1/4 -> CAN_EV/15  "<pBMSA_bool_DCChrgNegContaCmd>"
  Bus Selector1/5 -> CAN_EV/16  "<pBMSA_bool_DCChrgPosContaCmd>"
  Bus Selector1/6 -> CAN_EV/17  "<pTBCA_bool_BatChrgPerm>"
  Bus Selector1/7 -> CAN_EV/18  "<pTBCA_bool_BatHeatPerm>"
  Bus Selector1/8 -> CAN_EV/19  "<pDCCA_bool_DcDcCmd>"
  Bus Selector1/9 -> CAN_EV/20  "<pDCCA_V_DcDcOutUSp>"
  Bus Selector2/1 -> CAN_PT/1  "<pACPI_pct_AccPedVal>"
  Bus Selector2/2 -> CAN_PT/2  "<pBRPI_bool_BrkPedPrsd>"
  Bus Selector5/1 -> CAN_PT/3  "<pTMCA_bool_VechPermit>"
  Bus Selector5/2 -> CAN_PT/4  "<pTMCA_bool_IGOffReq>"
  Bus Selector5/3 -> CAN_PT/5  "<pTMCA_bool_AirCdnCmd>"
  Bus Selector5/4 -> CAN_PT/6  "<pTMCA_bool_BatCoolgReq>"
  Bus Selector5/5 -> CAN_PT/7  "<pSHLA_st_ShftLvrPosnIC>"
  Bus Selector5/6 -> CAN_PT/8  "<pSHLA_st_PrkgLock>"
  Bus Selector30/1 -> CAN_PT/9  "<pVMM_st_PtCoorrSts>"
  Bus Selector32/1 -> CAN_PT/10  "<pBMSI_A_BatActCurr>"
  Bus Selector32/2 -> CAN_PT/11  "<pTBCI_bool_ACChrgrPlugDtctd>"
  Bus Selector32/3 -> CAN_PT/12  "<pTBCI_bool_DCChrgrPlugDtctd>"
  Bus Selector32/4 -> CAN_PT/13  "<pBMSI_st_BMSChrgSt>"
  Bus Selector32/5 -> CAN_PT/14  "<pBMSI_pct_BatSOC>"
  Bus Selector32/6 -> CAN_PT/15  "<pSHLI_st_ECOSwtSt>"
  Bus Selector32/7 -> CAN_PT/16  "<pIGSI_st_OprtMode>"
  Bus Selector32/8 -> CAN_PT/17  "<pMCI_Nm_MCU1MotCtrlActTrq>"
  Bus Selector32/9 -> CAN_PT/18  "<pMCI_rpm_MCU1MotCtrlActRev>"
  Bus Selector32/10 -> CAN_PT/19  "<pMCI_rpm_MCU2MotCtrlActRev>"
  Bus Selector32/11 -> CAN_PT/20  "<pDCCI_V_DCDCOutVolt>"
  Bus Selector19/1 -> CAN_PT/21  "<pTMCA_bool_RemainACOnTip>"
  Bus Selector19/2 -> CAN_PT/22  "<pNMHA_bool_CanSlpCmd>"
  Bus Selector19/3 -> CAN_PT/23  "<pMCA_Nm_MCU1TMTorqReq>"
  Bus Selector19/4 -> CAN_PT/24  "<pMCA_Nm_MCU2TMTorqReq>"
  Bus Selector11/1 -> CAN_PT/25  "<pBMSI_st_BatIslaMeasSt>"
  Bus Selector11/2 -> CAN_PT/26  "<pDCCI_st_DCDCActSt>"
  Bus Selector11/3 -> CAN_PT/27  "<pBMSI_degC_BatAvgTemp>"
  Bus Selector11/4 -> CAN_PT/28  "<pBMSI_st_BMSErr>"
  Bus Selector11/5 -> CAN_PT/29  "<pBMSI_min_RemainChrgTime>"
  Bus Selector11/6 -> CAN_PT/30  "<pBMSI_kw_InstnsPwrCnsmp>"
  Bus Selector11/7 -> CAN_PT/31  "<pBMSI_V_BatActVolt>"
  Bus Selector3/1 -> CAN_PT/32  "<pACCA_bool_KickDwnReq>"
  Bus Selector3/2 -> CAN_PT/33  "<pACCA_bool_AccelPedOvrid>"
  Bus Selector3/3 -> CAN_PT/34  "<pACCA_pct_CalcAccelPedPstn>"
  Bus Selector3/4 -> CAN_PT/35  "<pACCA_bool_RespACC>"
  Bus Selector3/5 -> CAN_PT/36  "<pACCA_bool_CCMainSwt>"
  Bus Selector3/6 -> CAN_PT/37  "<pACCA_bool_CCCancelSwt>"
  Bus Selector3/7 -> CAN_PT/38  "<pACCA_bool_CCSetOrCoastSwt>"
  Bus Selector3/8 -> CAN_PT/39  "<pACCA_bool_HeadwaySwt>"
  Bus Selector3/9 -> CAN_PT/40  "<pACCA_bool_CCSwtErr>"
  Bus Selector3/10 -> CAN_PT/41  "<pACCA_bool_CCRsmOrAccelSwt>"
  Bus Selector3/11 -> CAN_PT/42  "<pACCA_Nm_ActDrvReqTrq>"
  Bus Selector3/12 -> CAN_PT/43  "<pACCA_Nm_MotMaxDrvTrq>"
  Bus Selector3/13 -> CAN_PT/44  "<pACCA_Nm_IndicateDrvPrimTrq>"
  Bus Selector3/14 -> CAN_PT/45  "<pACCA_Nm_IndicateDrvSecTrq>"
  Bus Selector4/1 -> CAN_PT/46  "<pESPA_Nm_MCU1ActBrkTrq>"
  Bus Selector4/2 -> CAN_PT/47  "<pESPA_Nm_MCU1MaxDrvTrq>"
  Bus Selector4/3 -> CAN_PT/48  "<pESPA_Nm_MCU1MaxGenrTrq>"
  Bus Selector4/4 -> CAN_PT/49  "<pESPA_Nm_MCU2ActBrkTrq>"
  Bus Selector4/5 -> CAN_PT/50  "<pESPA_Nm_MCU2MaxDrvTrq>"
  Bus Selector4/6 -> CAN_PT/51  "<pESPA_Nm_MCU2MaxGenrTrq>"
  CAN_PT/1 -> bus_CAN_PT/1
  CAN_PT/2 -> bus_CAN_PT/2
  CAN_PT/3 -> bus_CAN_PT/3
  CAN_PT/4 -> bus_CAN_PT/4
  CAN_PT/5 -> bus_CAN_PT/5
  CAN_PT/6 -> bus_CAN_PT/6
  CAN_PT/7 -> bus_CAN_PT/7
  CAN_PT/8 -> bus_CAN_PT/8
  CAN_PT/9 -> bus_CAN_PT/9
  CAN_PT/10 -> bus_CAN_PT/10
  CAN_PT/11 -> bus_CAN_PT/11
  CAN_PT/12 -> bus_CAN_PT/12
  CAN_PT/13 -> bus_CAN_PT/13
  CAN_PT/14 -> bus_CAN_PT/14
  CAN_PT/15 -> bus_CAN_PT/15
  CAN_PT/16 -> bus_CAN_PT/16
  CAN_PT/17 -> bus_CAN_PT/17
  CAN_PT/18 -> bus_CAN_PT/18
  CAN_PT/19 -> bus_CAN_PT/19
  CAN_PT/20 -> bus_CAN_PT/20
  CAN_PT/21 -> bus_CAN_PT/21
  CAN_PT/22 -> bus_CAN_PT/22
  CAN_PT/23 -> bus_CAN_PT/23
  CAN_PT/24 -> bus_CAN_PT/24
  CAN_PT/25 -> bus_CAN_PT/25
  CAN_PT/26 -> bus_CAN_PT/26
  CAN_PT/27 -> bus_CAN_PT/27
  CAN_PT/28 -> bus_CAN_PT/28
  CAN_PT/29 -> bus_CAN_PT/29
  CAN_PT/30 -> bus_CAN_PT/30
  CAN_PT/31 -> bus_CAN_PT/31
  CAN_PT/32 -> bus_CAN_PT/32
  CAN_PT/33 -> bus_CAN_PT/33
  CAN_PT/34 -> bus_CAN_PT/34
  CAN_PT/35 -> bus_CAN_PT/35
  CAN_PT/36 -> bus_CAN_PT/36
  CAN_PT/37 -> bus_CAN_PT/37
  CAN_PT/38 -> bus_CAN_PT/38
  CAN_PT/39 -> bus_CAN_PT/39
  CAN_PT/40 -> bus_CAN_PT/40
  CAN_PT/41 -> bus_CAN_PT/41
  CAN_PT/42 -> bus_CAN_PT/42
  CAN_PT/43 -> bus_CAN_PT/43
  CAN_PT/44 -> bus_CAN_PT/44
  CAN_PT/45 -> bus_CAN_PT/45
  CAN_PT/46 -> bus_CAN_PT/46
  CAN_PT/47 -> bus_CAN_PT/47
  CAN_PT/48 -> bus_CAN_PT/48
  CAN_PT/49 -> bus_CAN_PT/49
  CAN_PT/50 -> bus_CAN_PT/50
  CAN_PT/51 -> bus_CAN_PT/51
  CAN_PT/52 -> bus_CAN_PT/52
  CAN_PT/53 -> bus_CAN_PT/53
  CAN_PT/54 -> bus_CAN_PT/54
  CAN_PT/55 -> bus_CAN_PT/55
  CAN_PT/56 -> bus_CAN_PT/56
  CAN_PT/57 -> bus_CAN_PT/57
  CAN_PT/58 -> bus_CAN_PT/58
  CAN_PT/59 -> bus_CAN_PT/59
  CAN_PT/60 -> bus_CAN_PT/60
  CAN_PT/61 -> bus_CAN_PT/61
  CAN_PT/62 -> bus_CAN_PT/62
  CAN_PT/63 -> bus_CAN_PT/63
  Bus Selector6/1 -> CAN_PT/52  "<pESPI_ratio_AltitudeFac>"
